simulink library "AssessmentLibrary"  (R2015b)
settings: Solver=VariableStepAuto  StartTime=0.0  StopTime=10.0  RelTol=1e-3
settings Model: Creator=jdirner  LastModifiedBy=jdirner
settings HardwareCC: ProdWordSize=32
settings ModelReferenceCC: SkipRefExpFcnMdlSchedulingOrderCheck=off

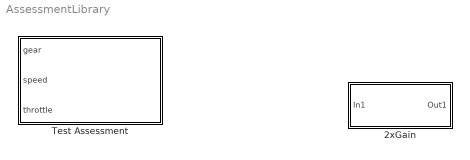
== system AssessmentLibrary ==
  2xGain : Subsystem
  Test Assessment : State Transition Table  TreatAsAtomicUnit=on

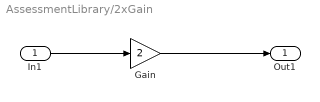
== system AssessmentLibrary/2xGain ==
  In1 : Inport
  Gain : Gain  Gain=2
  Out1 : Outport
  wires:
  In1/1 -> Gain/1
  Gain/1 -> Out1/1

== stateflow chart AssessmentLibrary/Test Assessment ==
  settings: stateMachineType=SIMPLIFIED_MACHINE
  state AssertConditions
    assert(speed >= 0);
    assert(throttle >= 0);
    assert(throttle <= 100);
    assert(gear > 0);
  (default) -> AssertConditions
  data: gear input; speed input; throttle input
